simulink model "sim_3"  (R2015b)
settings: Solver=ode23  StartTime=0  StopTime=1200  FixedStep=1e-3  RelTol=1e-4
undefined symbols (not defined in the file or in its folder): alpha_nc, alpha_nw, angle_AW, angle_current, angle_SW, currentCoeffMatrix, f, Kd_surge, Kd_sway, Kd_yaw, Ki_surge, Ki_sway, Ki_yaw, Kp_surge, Kp_sway, Kp_yaw, mu, mu_SW, N_freq, Par, phi, S, Sim, T_pinv, TA_sampling_time, thrusterPositionX, thrusterPositionY, thrusters, thrustersInitialAlpha, U_mean_AW, U_mean_c, U_mean_w, V_c, windCoeffMatrix
libraries: simulink_extras x5, simulink x5, marine_gnc x2
settings Model: Creator=torstebo  LastModifiedBy=ShivJeet
settings SolverCC: MaxConsecutiveMinStep=3  SolverJacobianMethodControl=FullPerturbation  ZeroCrossControl=DisableAll  ZeroCrossAlgorithm=Adaptive
settings DataIOCC: Decimation=10  InitialState=xFinal  LimitDataPoints=off  SaveFormat=StructureWithTime  SaveOutput=off  InspectSignalLogs=on  VisualizeSimOutput=off  SaveTime=off
settings OptimizationCC: AccelVerboseBuild=on
settings DebuggingCC: AlgebraicLoopMsg=error  UnderspecifiedInitializationDetection=Classic  MergeDetectMultiDrivingBlocksExec=none  SolverPrmCheckMsg=warning  StateNameClashWarn=warning
settings HardwareCC: ProdBitPerPointer=32  ProdLargestAtomicFloat=None  ProdIntDivRoundTo=Undefined  ProdEndianess=Unspecified  ProdWordSize=32  ProdHWDeviceType=32-bit Generic
settings GRTTargetCC: GeneratePreprocessorConditionals=Disable all
settings ConfigComp: CovModelRefEnable=Off  CovSFcnEnable=off

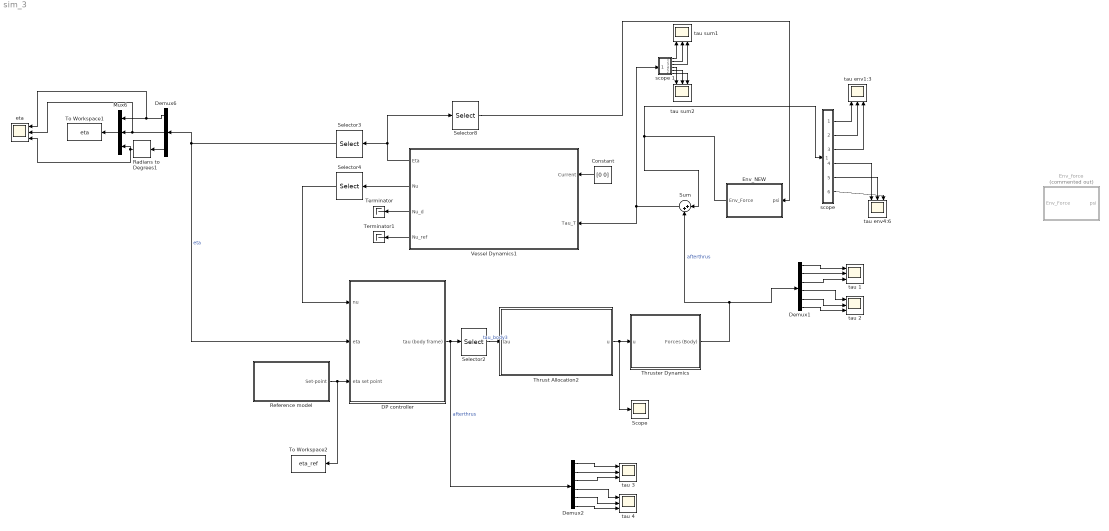
== system sim_3 ==
  Constant : Constant  Value=[0 0]
  DP controller : Subsystem
  Demux1 : Demux  Outputs=6
  Demux2 : Demux  Outputs=6
  Demux6 : Demux  Outputs=3
  Env_NEW : Subsystem
  Env_force : Subsystem  Commented=on
  Mux6 : Mux  Inputs=3
  Radians to Degrees1 : simulink_extras/Transformations/Radians to Degrees
  Reference model : Subsystem
  Scope : Scope
  Selector2 : Selector  InputPortWidth=6  IndexOptions=Index vector (dialog)  Indices=[1 2 6]  OutputSizes=1
  Selector3 : Selector  InputPortWidth=6  IndexOptions=Index vector (dialog)  Indices=[1 2 6]  OutputSizes=1
  Selector4 : Selector  InputPortWidth=6  IndexOptions=Index vector (dialog)  Indices=[1 2 6]  OutputSizes=1
  Selector8 : Selector  InputPortWidth=6  IndexOptions=Index vector (dialog)  Indices=[6]  OutputSizes=1
  Sum : Sum  Inputs=|++
  Terminator : Terminator
  Terminator1 : Terminator
  Thrust Allocation2 : Subsystem
  Thruster Dynamics : Subsystem  SystemSampleTime=TA_sampling_time  mask{wt=2, thrusterfault=off}
      mask prompts: wt "Thrusters Time constant"; thrusterfault "Thruster #3 fault?"
  To Workspace1 : ToWorkspace  VariableName=eta  SaveFormat=Timeseries  SampleTime=-1
  To Workspace2 : ToWorkspace  VariableName=eta_ref  SaveFormat=Timeseries  SampleTime=-1
  Vessel Dynamics1 : Subsystem
      mask Display:
      | image(imread('Files/supply.jpg'))
      | color('black'); port_label('output', 1, 'eta')
      | color('black'); port_label('output', 2, 'nu')
      | color('black'); port_label('output', 3, 'nu_d')
      | color('black'); port_label('output', 4, 'nu_ref')
      | color('black'); port_label('input', 1, 'nu_c')
      | color('black'); port_label('input', 2, 'tau')
  eta : Scope  NumInputPorts=3
  "scope " : Subsystem
  scope 1 : Subsystem
  tau {1..4} (4 alike) : Scope  NumInputPorts=3
  tau env1:3 : Scope  NumInputPorts=3
  tau env4:6 : Scope  NumInputPorts=3
  tau sum1 : Scope  NumInputPorts=3
  tau sum2 : Scope  NumInputPorts=3
  wires:
  Vessel Dynamics1/2(Nu) -> Selector4/1
  Constant/1 -> Vessel Dynamics1/1(Current)
  Reference model/1(Set-point) -> To Workspace2/1, DP controller/3(eta set point)
  Vessel Dynamics1/3(Nu_d) -> Terminator/1
  Thrust Allocation2/1(u) -> Scope/1, Thruster Dynamics/1(u)
  Selector4/1 -> DP controller/1(nu)
  Vessel Dynamics1/4(Nu_ref) -> Terminator1/1
  Thruster Dynamics/1(Forces (Body)) -> Sum/2, Demux1/1  "afterthrus"
  Selector3/1 -> Demux6/1, DP controller/2(eta)  "eta"
  Demux6/3 -> Radians to Degrees1/1
  Radians to Degrees1/1 -> Mux6/3, eta/3
  Demux6/2 -> eta/2, Mux6/2
  Demux6/1 -> Mux6/1, eta/1
  Mux6/1 -> To Workspace1/1
  Selector2/1 -> Thrust Allocation2/1(tau)  "tau_body3"
  Vessel Dynamics1/1(Eta) -> Selector3/1, Selector8/1
  Selector8/1 -> Env_NEW/1(psi)
  Sum/1 -> scope 1/1(In1), Vessel Dynamics1/2(Tau_T)
  Demux1/1 -> tau 1/1
  Demux1/2 -> tau 1/2
  Demux1/3 -> tau 1/3
  Demux1/4 -> tau 2/1
  Demux1/5 -> tau 2/2
  Demux1/6 -> tau 2/3
  Env_NEW/1(Env_Force) -> "scope "/1(In1), Sum/1
  "scope "/1(Out1) -> tau env1:3/1
  "scope "/3(Out3) -> tau env1:3/3
  "scope "/4(Out4) -> tau env4:6/1
  "scope "/5(Out5) -> tau env4:6/2
  "scope "/6(Out6) -> tau env4:6/3
  scope 1/1(Out1) -> tau sum1/1
  scope 1/2(Out2) -> tau sum1/2
  scope 1/3(Out3) -> tau sum1/3
  scope 1/4(Out4) -> tau sum2/1
  scope 1/5(Out5) -> tau sum2/2
  scope 1/6(Out6) -> tau sum2/3
  "scope "/2(Out2) -> tau env1:3/2
  DP controller/1(tau (body frame)) -> Demux2/1, Selector2/1  "afterthrus"
  Demux2/1 -> tau 3/1
  Demux2/2 -> tau 3/2
  Demux2/3 -> tau 3/3
  Demux2/4 -> tau 4/1
  Demux2/5 -> tau 4/2
  Demux2/6 -> tau 4/3

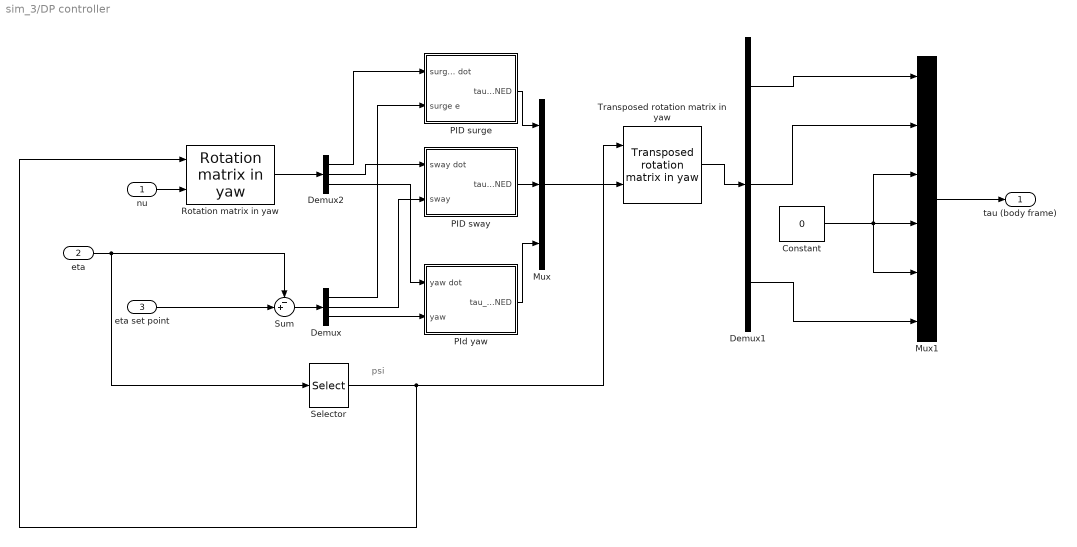
== system sim_3/DP controller ==
  note: psi
  nu : Inport
  eta : Inport  Port=2
  eta set point : Inport  Port=3
  Constant : Constant  Value=0
  Demux : Demux  Outputs=3
  Demux1 : Demux  Outputs=3
  Demux2 : Demux  Outputs=3
  Mux : Mux  Inputs=3
  Mux1 : Mux  Inputs=6
  PID surge : Subsystem
  PID sway : Subsystem
  "PId yaw " : Subsystem
  "Rotation matrix in yaw " : marine_gnc/Models/ Kinematics/Rotation matrix in yaw 
  Selector : Selector  InputPortWidth=3  IndexOptions=Index vector (dialog)  Indices=3  OutputSizes=1
  Sum : Sum  Inputs=-+|
  Transposed rotation matrix in yaw : marine_gnc/Models/ Kinematics/Transposed rotation  matrix in yaw
  tau (body frame) : Outport
  wires:
  Sum/1 -> Demux/1
  eta/1 -> Sum/1, Selector/1
  eta set point/1 -> Sum/2
  Demux2/1 -> PID surge/1(surge dot)
  Demux/1 -> PID surge/2(surge e)
  Demux2/2 -> PID sway/1(sway dot)
  Demux2/3 -> "PId yaw "/1(yaw dot)
  Demux/2 -> PID sway/2(sway)
  Demux/3 -> "PId yaw "/2(yaw)
  "PId yaw "/1(tau_yaw_NED) -> Mux/3
  PID surge/1(tau_surge_NED) -> Mux/1
  PID sway/1(tau_sway_NED) -> Mux/2
  nu/1 -> "Rotation matrix in yaw "/2
  Selector/1 -> Transposed rotation matrix in yaw/1, "Rotation matrix in yaw "/1
  "Rotation matrix in yaw "/1 -> Demux2/1
  Constant/1 -> Mux1/3, Mux1/4, Mux1/5
  Transposed rotation matrix in yaw/1 -> Demux1/1
  Demux1/1 -> Mux1/1
  Demux1/2 -> Mux1/2
  Demux1/3 -> Mux1/6
  Mux1/1 -> tau (body frame)/1
  ? -> ?
  Mux/1 -> Transposed rotation matrix in yaw/2

== system sim_3/Env_NEW ==
  psi : Inport
  Constant : Constant  Value=windCoeffMatrix
  Constant1 : Constant  Value=currentCoeffMatrix
  Current : Subsystem
  Product : Product  Inputs=3  RndMeth=Zero
  Product1 : Product  Inputs=3  RndMeth=Zero
  Radians to Degrees : simulink_extras/Transformations/Radians to Degrees
  Sum : Sum  Inputs=+-|
  Sum1 : Sum  Inputs=+|+
  Sum2 : Sum  Inputs=|+-
  Wind : Subsystem
  get current coeffcients : MATLAB Function  TreatAsAtomicUnit=on
  get wind coeffcients : MATLAB Function  TreatAsAtomicUnit=on
  Env_Force : Outport
  wires:
  Wind/1(Wind velocity) -> Product/2, Product/1
  Wind/2(Win direction) -> Sum/1
  psi/1 -> Radians to Degrees/1
  Sum1/1 -> Env_Force/1
  Current/1(current velocity) -> Product1/2, Product1/1
  Radians to Degrees/1 -> Sum/2, Sum2/2
  Current/2(current direction) -> Sum2/1
  Sum2/1 -> get current coeffcients/1(alpha)
  get current coeffcients/1(C) -> Product1/3
  Sum/1 -> get wind coeffcients/1(alpha)
  get wind coeffcients/1(C) -> Product/3
  Product1/1 -> Sum1/2
  Product/1 -> Sum1/1
  Constant/1 -> get wind coeffcients/2(windCoeffMatrix)
  Constant1/1 -> get current coeffcients/2(currentCoeffMatrix)

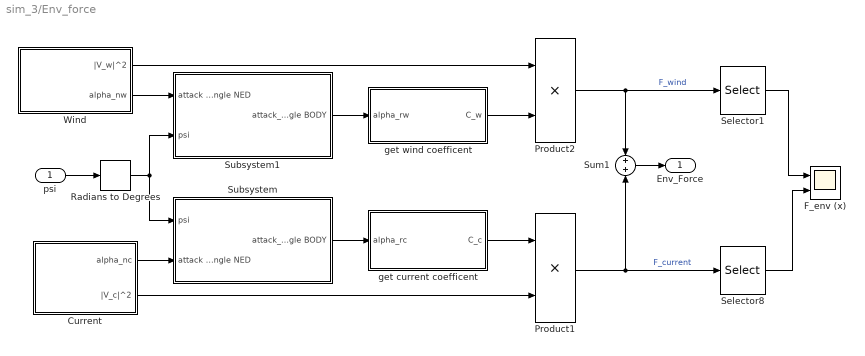
== system sim_3/Env_force ==
  psi : Inport
  "Current " : Subsystem
  F_env (x) : Scope  NumInputPorts=2
  Product1 : Product  RndMeth=Zero
  Product2 : Product  RndMeth=Zero
  Radians to Degrees : simulink_extras/Transformations/Radians to Degrees
  Selector1 : Selector  InputPortWidth=6  IndexOptions=Index vector (dialog)  Indices=[2]  OutputSizes=1
  Selector8 : Selector  InputPortWidth=6  IndexOptions=Index vector (dialog)  Indices=[2]  OutputSizes=1
  Subsystem : Subsystem
  Subsystem1 : Subsystem
  Sum1 : Sum  Inputs=+|+
  Wind : Subsystem
  "get current coefficent " : MATLAB Function  TreatAsAtomicUnit=on
  "get wind coefficent " : MATLAB Function  TreatAsAtomicUnit=on
  Env_Force : Outport
  wires:
  Wind/1(|V_w|^2) -> Product2/1
  psi/1 -> Radians to Degrees/1
  Sum1/1 -> Env_Force/1
  Product2/1 -> Selector1/1, Sum1/1  "F_wind"
  "Current "/2(|V_c|^2) -> Product1/2
  Product1/1 -> Selector8/1, Sum1/2  "F_current"
  Selector1/1 -> F_env (x)/1
  Selector8/1 -> F_env (x)/2
  "get current coefficent "/1(C_c) -> Product1/1
  Subsystem/1(attack_angle BODY) -> "get current coefficent "/1(alpha_rc)
  Radians to Degrees/1 -> Subsystem/1(psi), Subsystem1/2(psi)
  "Current "/1(alpha_nc) -> Subsystem/2(attack angle NED)
  Wind/2(alpha_nw) -> Subsystem1/1(attack angle NED)
  Subsystem1/1(attack_angle BODY) -> "get wind coefficent "/1(alpha_rw)
  "get wind coefficent "/1(C_w) -> Product2/2

== system sim_3/Reference model ==
  Mux : Mux  Inputs=3
  Sp_surge : Constant  Value=10*1  VectorParams1D=off
  Sp_sway : Constant  Value=2*1
  Sp_yaw : Constant  Value=pi/2*1
  Transfer Fcn1 : TransferFcn  Numerator=[0.05]  Denominator=[1 0.05]
  Transfer Fcn2 : TransferFcn  Numerator=[0.01]  Denominator=[1 0.01]
  Transfer Fcn3 : TransferFcn  Numerator=[0.05]  Denominator=[1 0.05]
  Set-point : Outport
  wires:
  Mux/1 -> Set-point/1
  Transfer Fcn1/1 -> Mux/1
  Transfer Fcn2/1 -> Mux/2
  Transfer Fcn3/1 -> Mux/3
  Sp_surge/1 -> Transfer Fcn1/1
  Sp_sway/1 -> Transfer Fcn2/1
  Sp_yaw/1 -> Transfer Fcn3/1

== system sim_3/Thrust Allocation2 ==
  tau : Inport
  Gain : Gain  Gain=T_pinv  Multiplication=Matrix(K*u) (u vector)
  u : Outport
  wires:
  tau/1 -> Gain/1
  Gain/1 -> u/1

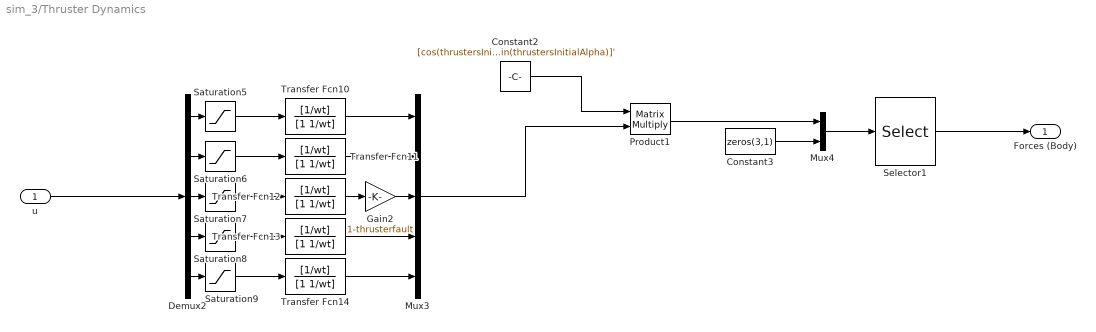
== system sim_3/Thruster Dynamics ==
  u : Inport  PortDimensions=[5 1]
  Constant2 : Constant  Value=[cos(thrustersInitialAlpha) sin(thrustersInitialAlpha) -thrusterPositionY.*cos(thrustersInitialAlpha)+thrusterPositionX.*sin(thrustersInitialAlpha)]'
  Constant3 : Constant  Value=zeros(3,1)
  Demux2 : Demux  Outputs=5
  Gain2 : Gain  Gain=1-thrusterfault
  Mux3 : Mux  Inputs=5
  Mux4 : Mux  Inputs=2
  Product1 : Product  Multiplication=Matrix(*)
  Saturation5 : Saturate  UpperLimit=thrusters(1).rated_thrust  LowerLimit=-thrusters(1).rated_thrust
  Saturation6 : Saturate  UpperLimit=thrusters(2).rated_thrust  LowerLimit=-thrusters(2).rated_thrust
  Saturation7 : Saturate  UpperLimit=thrusters(3).rated_thrust  LowerLimit=-thrusters(3).rated_thrust
  Saturation8 : Saturate  UpperLimit=thrusters(4).rated_thrust  LowerLimit=-thrusters(4).rated_thrust
  Saturation9 : Saturate  UpperLimit=thrusters(5).rated_thrust  LowerLimit=-thrusters(5).rated_thrust
  Selector1 : Selector  InputPortWidth=6  IndexOptions=Index vector (dialog)  Indices=[1 2 4 5 6 3]  OutputSizes=1
  Transfer Fcn{10..14} (5 alike) : TransferFcn  Numerator=[1/wt]  Denominator=[1 1/wt]
  Forces (Body) : Outport
  wires:
  Selector1/1 -> Forces (Body)/1
  Constant2/1 -> Product1/1
  Product1/1 -> Mux4/1
  Saturation5/1 -> Transfer Fcn10/1
  Demux2/1 -> Saturation5/1
  Demux2/2 -> Saturation6/1
  Saturation6/1 -> Transfer Fcn11/1
  Demux2/3 -> Saturation7/1
  Saturation7/1 -> Transfer Fcn12/1
  Demux2/4 -> Saturation8/1
  Saturation8/1 -> Transfer Fcn13/1
  Demux2/5 -> Saturation9/1
  Saturation9/1 -> Transfer Fcn14/1
  u/1 -> Demux2/1
  Transfer Fcn10/1 -> Mux3/1
  Transfer Fcn11/1 -> Mux3/2
  Transfer Fcn12/1 -> Gain2/1
  Transfer Fcn13/1 -> Mux3/4
  Transfer Fcn14/1 -> Mux3/5
  Mux4/1 -> Selector1/1
  Constant3/1 -> Mux4/2
  Gain2/1 -> Mux3/3
  Mux3/1 -> Product1/2

== system sim_3/Vessel Dynamics1 ==
  note: VESSEL MODULE
      | Consists of a WF and a LF module, which may be enabled or disabled in the Parameters file.
      | The LF and WFmotion components are written to the workspace for processing, and added for
      | use in the simulator.
  Current : Inport
  Tau_T : Inport  Port=2
  Vessel LF 6DOF : Subsystem
  Eta : Outport
  Nu : Outport  Port=2
  Nu_d : Outport  Port=3
  Nu_ref : Outport  Port=4
  wires:
  Current/1 -> Vessel LF 6DOF/2(Current_NED)
  Tau_T/1 -> Vessel LF 6DOF/1(External forces)  "Tau_T"
  Vessel LF 6DOF/1(Eta) -> Eta/1  "Eta_LF"
  Vessel LF 6DOF/2(Nu) -> Nu/1  "Nu_LF"
  Vessel LF 6DOF/3(Nu_d) -> Nu_d/1
  Vessel LF 6DOF/4(Nu_r) -> Nu_ref/1

== system sim_3/scope  ==
  In1 : Inport
  Demux2 : Demux  Outputs=6
  Out1 : Outport
  Out2 : Outport  Port=2
  Out3 : Outport  Port=3
  Out4 : Outport  Port=4
  Out5 : Outport  Port=5
  Out6 : Outport  Port=6
  wires:
  Demux2/2 -> Out2/1
  Demux2/1 -> Out1/1
  Demux2/5 -> Out5/1
  Demux2/4 -> Out4/1
  Demux2/6 -> Out6/1
  Demux2/3 -> Out3/1
  In1/1 -> Demux2/1

== system sim_3/scope 1 ==
  In1 : Inport
  Demux2 : Demux  Outputs=6
  Out1 : Outport
  Out2 : Outport  Port=2
  Out3 : Outport  Port=3
  Out4 : Outport  Port=4
  Out5 : Outport  Port=5
  Out6 : Outport  Port=6
  wires:
  Demux2/2 -> Out2/1
  Demux2/1 -> Out1/1
  Demux2/5 -> Out5/1
  Demux2/4 -> Out4/1
  Demux2/6 -> Out6/1
  Demux2/3 -> Out3/1
  In1/1 -> Demux2/1

== system sim_3/DP controller/PID surge ==
  surge dot : Inport
  surge e : Inport  Port=2
  Gain2 : Gain  Gain=Ki_surge
  Integrator : Integrator
  KP : Gain  Gain=Kp_surge
  Kd : Gain  Gain=Kd_surge
  Sum : Sum  Inputs=|-++
  tau_surge_NED : Outport
  wires:
  surge dot/1 -> Kd/1
  surge e/1 -> KP/1, Integrator/1
  Integrator/1 -> Gain2/1
  Kd/1 -> Sum/1
  KP/1 -> Sum/2
  Gain2/1 -> Sum/3
  Sum/1 -> tau_surge_NED/1

== system sim_3/DP controller/PID sway ==
  sway dot : Inport
  sway : Inport  Port=2
  Integrator : Integrator
  Kd : Gain  Gain=Kd_sway
  Ki : Gain  Gain=Ki_sway
  Kp : Gain  Gain=Kp_sway
  Sum : Sum  Inputs=|-++
  tau_sway_NED : Outport
  wires:
  sway dot/1 -> Kd/1
  sway/1 -> Kp/1, Integrator/1
  Integrator/1 -> Ki/1
  Kd/1 -> Sum/1
  Kp/1 -> Sum/2
  Ki/1 -> Sum/3
  Sum/1 -> tau_sway_NED/1

== system sim_3/DP controller/PId yaw  ==
  yaw dot : Inport
  yaw : Inport  Port=2
  Gain : Gain  Gain=Kd_yaw
  Gain1 : Gain  Gain=Kp_yaw
  Gain2 : Gain  Gain=Ki_yaw
  Integrator : Integrator
  Sum : Sum  Inputs=|-++
  tau_yaw_NED : Outport
  wires:
  yaw dot/1 -> Gain/1
  yaw/1 -> Gain1/1, Integrator/1
  Integrator/1 -> Gain2/1
  Gain/1 -> Sum/1
  Gain1/1 -> Sum/2
  Gain2/1 -> Sum/3
  Sum/1 -> tau_yaw_NED/1

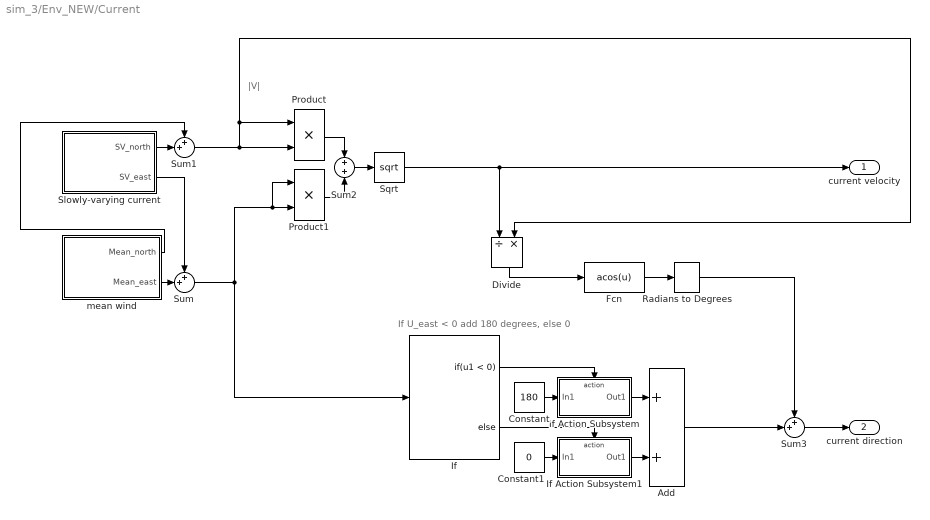
== system sim_3/Env_NEW/Current ==
  note: If U_east < 0 add 180 degrees, else 0
  note: |V|
  Add : Sum
  Constant : Constant  Value=180
  Constant1 : Constant  Value=0
  Divide : Product  Inputs=/*
  Fcn : Fcn  Expr=acos(u)
  "If " : If  IfExpression=u1 < 0
  If Action Subsystem : Subsystem  TreatAsAtomicUnit=on
  If Action Subsystem1 : Subsystem  TreatAsAtomicUnit=on
  Product : Product
  Product1 : Product
  Radians to Degrees : simulink_extras/Transformations/Radians to Degrees
  Slowly-varying current : Subsystem
  Sqrt : Sqrt  SaturateOnIntegerOverflow=on
  Sum : Sum  Inputs=++|
  Sum1 : Sum  Inputs=++|
  Sum2 : Sum  Inputs=+|+
  Sum3 : Sum  Inputs=++|
  mean wind : Subsystem
  current velocity : Outport
  current direction : Outport  Port=2
  wires:
  Slowly-varying current/1(SV_north) -> Sum1/2
  Slowly-varying current/2(SV_east) -> Sum/1
  mean wind/2(Mean_east) -> Sum/2
  Divide/1 -> Fcn/1
  Fcn/1 -> Radians to Degrees/1
  Sum3/1 -> current direction/1
  Radians to Degrees/1 -> Sum3/1
  If Action Subsystem/1(Out1) -> Add/1
  Add/1 -> Sum3/2
  mean wind/1(Mean_north) -> Sum1/1
  Sum1/1 -> Product/2, Product/1, Divide/2
  Sum/1 -> Product1/1, Product1/2, "If "/1
  Product/1 -> Sum2/1
  Product1/1 -> Sum2/2
  Sum2/1 -> Sqrt/1
  Sqrt/1 -> Divide/1, current velocity/1
  Constant/1 -> If Action Subsystem/1(In1)
  "If "/1 -> If Action Subsystem/Action
  "If "/2 -> If Action Subsystem1/Action
  Constant1/1 -> If Action Subsystem1/1(In1)
  If Action Subsystem1/1(Out1) -> Add/2

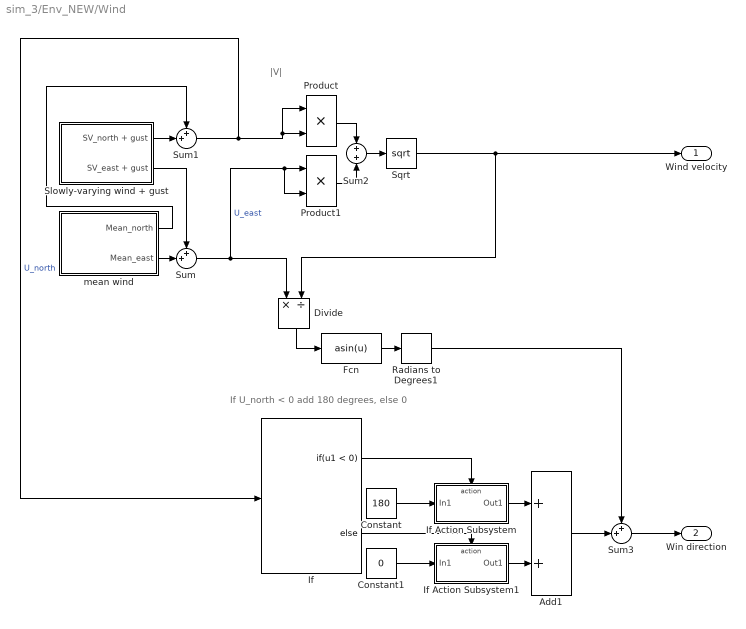
== system sim_3/Env_NEW/Wind ==
  note: |V|
  note: If U_north < 0 add 180 degrees, else 0
  Add1 : Sum
  Constant : Constant  Value=180
  Constant1 : Constant  Value=0
  Divide : Product  Inputs=*/
  Fcn : Fcn  Expr=asin(u)
  If : If  IfExpression=u1 < 0
  If Action Subsystem : Subsystem  TreatAsAtomicUnit=on
  If Action Subsystem1 : Subsystem  TreatAsAtomicUnit=on
  Product : Product
  Product1 : Product
  Radians to Degrees1 : simulink_extras/Transformations/Radians to Degrees
  Slowly-varying wind + gust : Subsystem
  Sqrt : Sqrt  SaturateOnIntegerOverflow=on
  Sum : Sum  Inputs=++|
  Sum1 : Sum  Inputs=++|
  Sum2 : Sum  Inputs=+|+
  Sum3 : Sum  Inputs=++|
  mean wind : Subsystem
  Wind velocity : Outport
  Win direction : Outport  Port=2
  wires:
  Slowly-varying wind + gust/2(SV_east + gust) -> Sum/1
  mean wind/2(Mean_east) -> Sum/2
  Sum1/1 -> Product/1, Product/2, If/1  "U_north"
  Sum/1 -> Product1/2, Product1/1, Divide/1  "U_east"
  Sqrt/1 -> Divide/2, Wind velocity/1
  Slowly-varying wind + gust/1(SV_north + gust) -> Sum1/2
  mean wind/1(Mean_north) -> Sum1/1
  Product/1 -> Sum2/1
  Product1/1 -> Sum2/2
  Sum2/1 -> Sqrt/1
  Divide/1 -> Fcn/1
  Fcn/1 -> Radians to Degrees1/1
  Radians to Degrees1/1 -> Sum3/1
  Add1/1 -> Sum3/2
  Sum3/1 -> Win direction/1
  If Action Subsystem/1(Out1) -> Add1/1
  Constant/1 -> If Action Subsystem/1(In1)
  If/1 -> If Action Subsystem/Action
  If/2 -> If Action Subsystem1/Action
  Constant1/1 -> If Action Subsystem1/1(In1)
  If Action Subsystem1/1(Out1) -> Add1/2

== system sim_3/Env_force/Current  ==
  Product : Product
  alpha current : Constant  Value=angle_current
  current speed : Constant  Value=V_c
  alpha_nc : Outport
  |V_c|^2 : Outport  Port=2
  wires:
  current speed/1 -> Product/2, Product/1
  alpha current/1 -> alpha_nc/1
  Product/1 -> |V_c|^2/1

== system sim_3/Env_force/Subsystem ==
  psi : Inport
  attack angle NED : Inport  Port=2
  Constant1 : Constant  Value=180
  Sum1 : Sum  Inputs=++-|
  attack_angle BODY : Outport
  wires:
  attack angle NED/1 -> Sum1/3
  Constant1/1 -> Sum1/1
  Sum1/1 -> attack_angle BODY/1
  psi/1 -> Sum1/2

== system sim_3/Env_force/Subsystem1 ==
  attack angle NED : Inport
  psi : Inport  Port=2
  Constant : Constant  Value=180
  Sum2 : Sum  Inputs=++-|
  attack_angle BODY : Outport
  wires:
  attack angle NED/1 -> Sum2/3
  Constant/1 -> Sum2/1
  Sum2/1 -> attack_angle BODY/1
  psi/1 -> Sum2/2

== system sim_3/Env_force/Wind ==
  Divide : Product  Inputs=/*
  Product : Product
  Slowly-varying wind : Subsystem
  Sum : Sum  Inputs=|++
  Sum1 : Sum  Inputs=++|
  average wind : Subsystem
  |V_w|^2 : Outport
  alpha_nw : Outport  Port=2
  wires:
  Slowly-varying wind/1(U_sv) -> Sum/1
  Sum/1 -> Product/1, Divide/1, Product/2
  Sum1/1 -> Divide/2
  Divide/1 -> alpha_nw/1
  average wind/2(wheigted direction) -> Sum1/1
  Slowly-varying wind/2(weigthed direction) -> Sum1/2
  average wind/1(speed) -> Sum/2
  Product/1 -> |V_w|^2/1

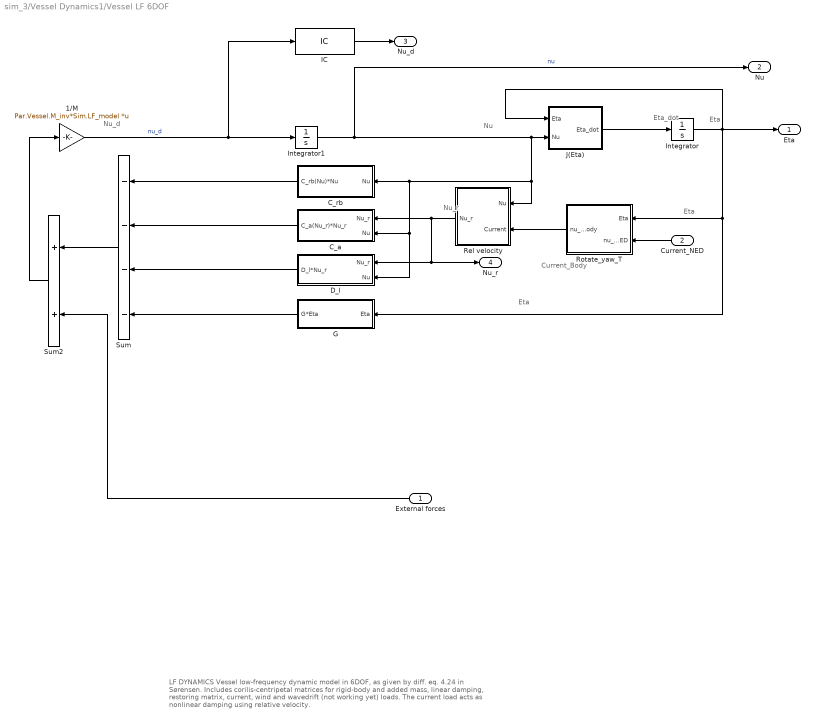
== system sim_3/Vessel Dynamics1/Vessel LF 6DOF ==
  note: Nu_d
  note: Nu
  note: Eta
  note: Current_Body
  note: Eta
  note: Nu_r
  note: Eta
  note: LF DYNAMICS
      | Vessel low-frequency dynamic model in 6DOF, as given by diff. eq. 4.24 in Sørensen.
      | Includes corilis-centripetal matrices for rigid-body and added mass, linear damping,
      | restoring matrix, current, wind and wavedrift (not working yet) loads. The current load
      | acts as nonlinear damping using relative velocity.
  note: Eta_dot
  External forces : Inport
  Current_NED : Inport  Port=2
  1/M : Gain  Gain=Par.Vessel.M_inv*Sim.LF_model  Multiplication=Matrix(K*u) (u vector)  SaturateOnIntegerOverflow=on  OutDataTypeStr=Inherit: Same as input  ParamDataTypeStr=Inherit: Same as input
  C_a : Subsystem
  C_rb : Subsystem
  D_l : Subsystem
      settings: MinAlgLoopOccurrences=on
  G : Subsystem
  IC : InitialCondition  Value=Sim.Nu_d_init
  Integrator : Integrator  InitialCondition=Sim.Eta_init
  Integrator1 : Integrator  InitialCondition=Sim.Nu_init
  J(Eta) : Subsystem
  Rel velocity : Subsystem
  Rotate_yaw_T : Subsystem
  Sum : Sum  Inputs=----  SaturateOnIntegerOverflow=on
  Sum2 : Sum  SaturateOnIntegerOverflow=on
  Eta : Outport
  Nu : Outport  Port=2
  Nu_d : Outport  Port=3
  Nu_r : Outport  Port=4
  wires:
  1/M/1 -> IC/1, Integrator1/1  "nu_d"
  J(Eta)/1(Eta_dot) -> Integrator/1
  Integrator/1 -> J(Eta)/1(Eta), Eta/1, Rotate_yaw_T/1(Eta), G/1(Eta)
  Integrator1/1 -> Nu/1, J(Eta)/2(Nu), Rel velocity/1(Nu), C_a/2(Nu), D_l/2(Nu), C_rb/1(Nu)  "nu"
  Current_NED/1 -> Rotate_yaw_T/2(nu_2D_NED)
  Rotate_yaw_T/1(nu_2D_body) -> Rel velocity/2(Current)
  Rel velocity/1(Nu_r) -> D_l/1(Nu_r), Nu_r/1, C_a/1(Nu_r)
  Sum/1 -> Sum2/1
  External forces/1 -> Sum2/2
  Sum2/1 -> 1/M/1
  C_rb/1(C_rb(Nu)*Nu) -> Sum/1
  C_a/1(C_a(Nu_r)*Nu_r) -> Sum/2
  D_l/1(D_l*Nu_r) -> Sum/3
  G/1(G*Eta) -> Sum/4
  IC/1 -> Nu_d/1

== system sim_3/Env_NEW/Current/If Action Subsystem ==
  In1 : Inport
  Action Port : ActionPort  ActionType=then
  Out1 : Outport
  wires:
  In1/1 -> Out1/1

== system sim_3/Env_NEW/Current/If Action Subsystem1 ==
  In1 : Inport
  Action Port : ActionPort  ActionType=else
  Out1 : Outport
  wires:
  In1/1 -> Out1/1

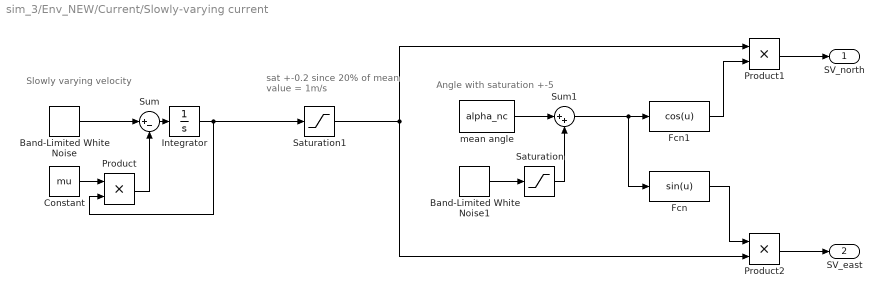
== system sim_3/Env_NEW/Current/Slowly-varying current ==
  note: Angle with saturation +-5
  note: Slowly varying velocity
  note: sat +-0.2 since 20%
      | of mean value = 1m/s
  Band-Limited White Noise : simulink/Sources/Band-Limited White Noise  Cov=[0.00005]  Ts=20  seed=[23343]
  Band-Limited White Noise1 : simulink/Sources/Band-Limited White Noise  Cov=[0.00005]  Ts=20  seed=[23344]
  Constant : Constant  Value=mu
  Fcn : Fcn  Expr=sin(u)
  Fcn1 : Fcn  Expr=cos(u)
  Integrator : Integrator
  Product : Product  RndMeth=Zero
  Product1 : Product  RndMeth=Zero
  Product2 : Product  RndMeth=Zero
  Saturation : Saturate  UpperLimit=(5*pi)/180  LowerLimit=-(5*pi)/180
  Saturation1 : Saturate  UpperLimit=0.2  LowerLimit=-0.2
  Sum : Sum  Inputs=|+-
  Sum1 : Sum  Inputs=|++
  mean angle : Constant  Value=alpha_nc
  SV_north : Outport
  SV_east : Outport  Port=2
  wires:
  Band-Limited White Noise/1 -> Sum/1
  Sum/1 -> Integrator/1
  Integrator/1 -> Product/2, Saturation1/1
  Product/1 -> Sum/2
  Constant/1 -> Product/1
  Fcn1/1 -> Product1/2
  mean angle/1 -> Sum1/1
  Sum1/1 -> Fcn/1, Fcn1/1
  Saturation/1 -> Sum1/2
  Band-Limited White Noise1/1 -> Saturation/1
  Product1/1 -> SV_north/1
  Product2/1 -> SV_east/1
  Saturation1/1 -> Product2/2, Product1/1
  Fcn/1 -> Product2/1

== system sim_3/Env_NEW/Current/mean wind ==
  Constant : Constant  Value=U_mean_c
  Fcn : Fcn  Expr=sin(u)
  Fcn1 : Fcn  Expr=cos(u)
  Product1 : Product  RndMeth=Zero
  Product2 : Product  RndMeth=Zero
  meen wind : Constant  Value=alpha_nc
  Mean_north : Outport
  Mean_east : Outport  Port=2
  wires:
  Constant/1 -> Product1/1, Product2/2
  Fcn1/1 -> Product1/2
  Product1/1 -> Mean_north/1
  Product2/1 -> Mean_east/1
  meen wind/1 -> Fcn/1, Fcn1/1
  Fcn/1 -> Product2/1

== system sim_3/Env_NEW/Wind/If Action Subsystem ==
  In1 : Inport
  Action Port : ActionPort  ActionType=then
  Out1 : Outport
  wires:
  In1/1 -> Out1/1

== system sim_3/Env_NEW/Wind/If Action Subsystem1 ==
  In1 : Inport
  Action Port : ActionPort  ActionType=else
  Out1 : Outport
  wires:
  In1/1 -> Out1/1

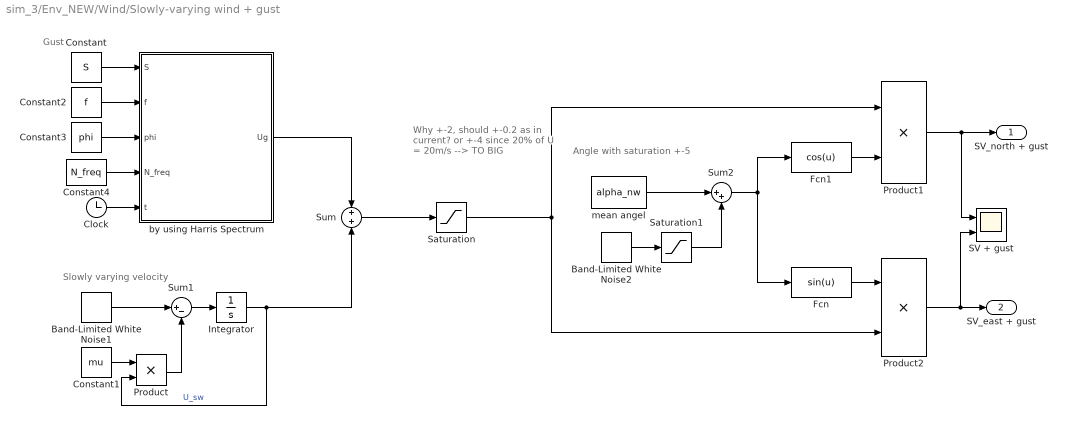
== system sim_3/Env_NEW/Wind/Slowly-varying wind + gust ==
  note: Gust
  note: Slowly varying velocity
  note: Angle with saturation +-5
  note: Why +-2, should
      | +-0.2 as in current?
      | or +-4 since 20% of
      | U = 20m/s --> TO BIG
  Band-Limited White Noise1 : simulink/Sources/Band-Limited White Noise  Cov=[0.005]  Ts=20  seed=[23341]
  Band-Limited White Noise2 : simulink/Sources/Band-Limited White Noise  Cov=[0.005]  Ts=20  seed=[23342]
  Clock : Clock
  Constant : Constant  Value=S
  Constant1 : Constant  Value=mu
  Constant2 : Constant  Value=f
  Constant3 : Constant  Value=phi
  Constant4 : Constant  Value=N_freq
  Fcn : Fcn  Expr=sin(u)
  Fcn1 : Fcn  Expr=cos(u)
  Integrator : Integrator
  Product : Product  RndMeth=Zero
  Product1 : Product  RndMeth=Zero
  Product2 : Product  RndMeth=Zero
  SV + gust : Scope  NumInputPorts=2
  Saturation : Saturate  UpperLimit=2  LowerLimit=-2
  Saturation1 : Saturate  UpperLimit=(5*pi)/180  LowerLimit=-(5*pi)/180
  Sum : Sum  Inputs=+|+
  Sum1 : Sum  Inputs=|+-
  Sum2 : Sum  Inputs=|++
  by using Harris Spectrum : MATLAB Function  TreatAsAtomicUnit=on  SystemSampleTime=1
  mean angel : Constant  Value=alpha_nw
  SV_north + gust : Outport
  SV_east + gust : Outport  Port=2
  wires:
  Fcn1/1 -> Product1/2
  Product1/1 -> SV + gust/1, SV_north + gust/1
  Product2/1 -> SV_east + gust/1, SV + gust/2
  Sum2/1 -> Fcn/1, Fcn1/1
  Integrator/1 -> Sum/2, Product/2  "U_sw"
  Saturation/1 -> Product1/1, Product2/2
  Constant1/1 -> Product/1
  Sum1/1 -> Integrator/1
  Product/1 -> Sum1/2
  Band-Limited White Noise1/1 -> Sum1/1
  mean angel/1 -> Sum2/1
  Saturation1/1 -> Sum2/2
  Band-Limited White Noise2/1 -> Saturation1/1
  Fcn/1 -> Product2/1
  Constant/1 -> by using Harris Spectrum/1(S)
  Constant2/1 -> by using Harris Spectrum/2(f)
  Constant3/1 -> by using Harris Spectrum/3(phi)
  Constant4/1 -> by using Harris Spectrum/4(N_freq)
  Clock/1 -> by using Harris Spectrum/5(t)
  Sum/1 -> Saturation/1
  by using Harris Spectrum/1(Ug) -> Sum/1

== system sim_3/Env_NEW/Wind/mean wind ==
  Constant : Constant  Value=U_mean_w
  Fcn : Fcn  Expr=sin(u)
  Fcn1 : Fcn  Expr=cos(u)
  Product1 : Product  RndMeth=Zero
  Product2 : Product  RndMeth=Zero
  mean wind : Constant  Value=alpha_nw
  Mean_north : Outport
  Mean_east : Outport  Port=2
  wires:
  Constant/1 -> Product2/2, Product1/1
  Fcn1/1 -> Product1/2
  Product1/1 -> Mean_north/1
  mean wind/1 -> Fcn1/1, Fcn/1
  Fcn/1 -> Product2/1
  Product2/1 -> Mean_east/1

== system sim_3/Env_force/Wind/Slowly-varying wind ==
  " angle SW" : Constant  Value=angle_SW
  Band-Limited White Noise : simulink/Sources/Band-Limited White Noise  Cov=white_noise_power_SW  Ts=1  seed=[23341]
  Constant : Constant  Value=mu_SW
  Integrator : Integrator
  Product : Product  RndMeth=Zero
  Product1 : Product  RndMeth=Zero
  Sum : Sum  Inputs=|+-
  U_sv : Outport
  weigthed direction : Outport  Port=2
  wires:
  Band-Limited White Noise/1 -> Sum/1
  Sum/1 -> Integrator/1
  Integrator/1 -> Product/2, U_sv/1, Product1/1
  Product/1 -> Sum/2
  Constant/1 -> Product/1
  Product1/1 -> weigthed direction/1
  " angle SW"/1 -> Product1/2

== system sim_3/Env_force/Wind/average wind ==
  Product : Product  RndMeth=Zero
  U_mean : Constant  Value=U_mean_AW
  wind angle : Constant  Value=angle_AW
  speed : Outport
  wheigted direction : Outport  Port=2
  wires:
  U_mean/1 -> speed/1, Product/1
  wind angle/1 -> Product/2
  Product/1 -> wheigted direction/1

== system sim_3/Vessel Dynamics1/Vessel LF 6DOF/C_a ==
  note: C_a
      | Coriolis-centripetal added mass force calculation using the S-function m2c_S.
      | This effect can be included/excluded from the Parameters file.
      | A choice of using absolute or relative vessel velocity is also given.
      | OS2002
  Nu_r : Inport
  Nu : Inport  Port=2
  C_a calculation : Subsystem  TreatAsAtomicUnit=on
  Enable Coriolis added mass force : Constant  Value=Sim.C_a
  Sim.Nu_r_C_a : Constant  Value=Sim.Nu_r_C_a
  Switch : Switch  Criteria=u2 > Threshold  SaturateOnIntegerOverflow=on
  C_a(Nu_r)*Nu_r : Outport
  wires:
  C_a calculation/1(F) -> C_a(Nu_r)*Nu_r/1
  Nu_r/1 -> Switch/1
  Nu/1 -> Switch/3
  Sim.Nu_r_C_a/1 -> Switch/2
  Switch/1 -> C_a calculation/1(Nu_r)
  Enable Coriolis added mass force/1 -> C_a calculation/Enable

== system sim_3/Vessel Dynamics1/Vessel LF 6DOF/C_rb ==
  note: C_rb
      | Coriolis-centripetal rigid-body force calculation using the S-function m2c_S.
      | This effect can be included/excluded from the Parameters file.
      | OS2002
  Nu : Inport
  C_rb Calculation : Subsystem  TreatAsAtomicUnit=on
  Enable Coriolis added mass force : Constant  Value=Sim.C_rb
  C_rb(Nu)*Nu : Outport
  wires:
  Nu/1 -> C_rb Calculation/1(Nu_r)
  Enable Coriolis added mass force/1 -> C_rb Calculation/Enable
  C_rb Calculation/1(F) -> C_rb(Nu)*Nu/1

== system sim_3/Vessel Dynamics1/Vessel LF 6DOF/D_l ==
  note: D_l
      | Linear damping, matrix formulation.
      | This effect can be included/excluded from the Parameters file.
      | A choice of using absolute or relative vessel velocity is also given.
      | OS2002
  Nu_r : Inport
  Nu : Inport  Port=2
  D_l : Gain  Gain=Par.Vessel.DL  Multiplication=Matrix(K*u)  SaturateOnIntegerOverflow=on  OutDataTypeStr=Inherit: Same as input  ParamDataTypeStr=Inherit: Same as input
  Include D_l : Gain  Gain=Sim.D_l  SaturateOnIntegerOverflow=on  OutDataTypeStr=Inherit: Same as input  ParamDataTypeStr=Inherit: Same as input
  Sim.Nu_r_D_l : Constant  Value=Sim.Nu_r_D_l
  Switch : Switch  Criteria=u2 > Threshold  SaturateOnIntegerOverflow=on
  D_l*Nu_r : Outport
  wires:
  D_l/1 -> Include D_l/1
  Include D_l/1 -> D_l*Nu_r/1
  Switch/1 -> D_l/1
  Nu_r/1 -> Switch/1
  Nu/1 -> Switch/3
  Sim.Nu_r_D_l/1 -> Switch/2

== system sim_3/Vessel Dynamics1/Vessel LF 6DOF/G ==
  note: G
      | Standard restoring matrix. This effect can
      | be included/excluded from the Parameters file.
      | OS2002
  Eta : Inport
  G : Gain  Gain=Par.Vessel.G  Multiplication=Matrix(K*u)  SaturateOnIntegerOverflow=on  OutDataTypeStr=Inherit: Same as input  ParamDataTypeStr=Inherit: Same as input
  Include G : Gain  Gain=Sim.G  SaturateOnIntegerOverflow=on  OutDataTypeStr=Inherit: Same as input  ParamDataTypeStr=Inherit: Same as input
  G*Eta : Outport
  wires:
  Eta/1 -> G/1
  G/1 -> Include G/1
  Include G/1 -> G*Eta/1

== system sim_3/Vessel Dynamics1/Vessel LF 6DOF/J(Eta) ==
  note: Theta
  note: v
  note: omega
  note: J(Eta)
      | Standard 6DOF rotation matrix, as defined by Fossen. Using the two
      | rotation matrices Rnb and Tnb from the gnc Simulink toolbox.
      | OS2002
  Eta : Inport
  Nu : Inport  Port=2
  Mux : Mux  Inputs=2
  Product : Product  Inputs=**  Multiplication=Matrix(*)  SaturateOnIntegerOverflow=on  OutDataTypeStr=Inherit: Same as first input
  Product1 : Product  Inputs=**  Multiplication=Matrix(*)  SaturateOnIntegerOverflow=on  OutDataTypeStr=Inherit: Same as first input
  Rnb_gnc : Subsystem
  Selector : Selector  InputPortWidth=6  IndexOptions=Index vector (dialog)  Indices=[4 5 6]  OutputSizes=1
  Selector1 : Selector  InputPortWidth=6  IndexOptions=Index vector (dialog)  Indices=[1 2 3]  OutputSizes=1
  Selector2 : Selector  InputPortWidth=6  IndexOptions=Index vector (dialog)  Indices=[4 5 6]  OutputSizes=1
  Tnb_gnc : Subsystem
  Eta_dot : Outport
  wires:
  Selector/1 -> Tnb_gnc/1(theta), Rnb_gnc/1(theta)
  Eta/1 -> Selector/1
  Rnb_gnc/1(Rzyx) -> Product/1
  Nu/1 -> Selector1/1, Selector2/1
  Selector1/1 -> Product/2
  Selector2/1 -> Product1/2
  Tnb_gnc/1(T) -> Product1/1
  Product/1 -> Mux/1
  Mux/1 -> Eta_dot/1
  Product1/1 -> Mux/2

== system sim_3/Vessel Dynamics1/Vessel LF 6DOF/Rel velocity ==
  note: REL VELOCITY
      | Calculate relative vessel velociy
      | including current.
      | OS2002
  Nu : Inport
  Current : Inport  Port=2
  Mux : Mux  Inputs=2
  Sum : Sum  Inputs=+-  SaturateOnIntegerOverflow=on
  Zeros : Constant  Value=[0 0 0 0]
  Nu_r : Outport
  wires:
  Current/1 -> Mux/1
  Nu/1 -> Sum/1
  Sum/1 -> Nu_r/1
  Mux/1 -> Sum/2
  Zeros/1 -> Mux/2

== system sim_3/Vessel Dynamics1/Vessel LF 6DOF/Rotate_yaw_T ==
  note: ROTATE_YAW_T
      | The transposed rotation matrix in yaw, as defined
      | by Fossen. Rotates a velocity or coordinate a positive
      | yaw angle. Corresponds to matlab function  rotate_yaw_T
      | by OS. Uses the gcn Simulink function GNC: "Transposed
      | rotation matrix yaw"
      | OS2002
  Eta : Inport
  nu_2D_NED : Inport  Port=2
  "GNC: \"Transposed rotation matrix yaw\"" : Subsystem
  Mux : Mux  Inputs=2
  Selector : Selector  InputPortWidth=3  IndexOptions=Index vector (dialog)  Indices=[1 2]  OutputSizes=1
  Selector1 : Selector  InputPortWidth=6  IndexOptions=Index vector (dialog)  Indices=6  OutputSizes=1
  psi : Constant  Value=0
  nu_2D_body : Outport
  wires:
  Selector1/1 -> "GNC: \"Transposed rotation matrix yaw\""/1(psi)
  nu_2D_NED/1 -> Mux/1
  psi/1 -> Mux/2
  "GNC: \"Transposed rotation matrix yaw\""/1(R*nu) -> Selector/1
  Selector/1 -> nu_2D_body/1
  Eta/1 -> Selector1/1
  Mux/1 -> "GNC: \"Transposed rotation matrix yaw\""/2(nu)

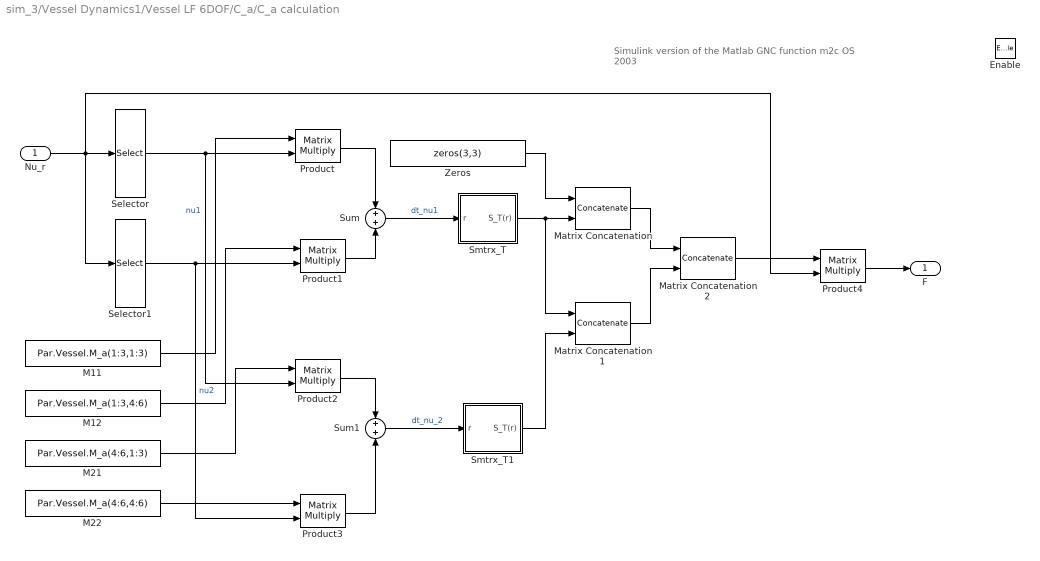
== system sim_3/Vessel Dynamics1/Vessel LF 6DOF/C_a/C_a calculation ==
  note: Simulink version of the Matlab GNC function m2c
      | OS 2003
  Nu_r : Inport
  Enable : EnablePort
  M11 : Constant  Value=Par.Vessel.M_a(1:3,1:3)
  M12 : Constant  Value=Par.Vessel.M_a(1:3,4:6)
  M21 : Constant  Value=Par.Vessel.M_a(4:6,1:3)
  M22 : Constant  Value=Par.Vessel.M_a(4:6,4:6)
  Matrix Concatenation : Concatenate  Mode=Multidimensional array  ConcatenateDimension=2
  Matrix Concatenation1 : Concatenate  Mode=Multidimensional array  ConcatenateDimension=2
  Matrix Concatenation2 : Concatenate  Mode=Multidimensional array
  Product{,1..4} (5 alike) : Product  Multiplication=Matrix(*)  SaturateOnIntegerOverflow=on  OutDataTypeStr=Inherit: Same as first input
  Selector : Selector  InputPortWidth=6  IndexOptions=Index vector (dialog)  Indices=[1:3]  OutputSizes=1
  Selector1 : Selector  InputPortWidth=6  IndexOptions=Index vector (dialog)  Indices=[4:6]  OutputSizes=1
  Smtrx_T : Subsystem
  Smtrx_T1 : Subsystem
  Sum : Sum  Inputs=+|+  SaturateOnIntegerOverflow=on
  Sum1 : Sum  Inputs=+|+  SaturateOnIntegerOverflow=on
  Zeros : Constant  Value=zeros(3,3)
  F : Outport
  wires:
  Nu_r/1 -> Selector/1, Selector1/1, Product4/2
  Product/1 -> Sum/1
  Product1/1 -> Sum/2
  Product2/1 -> Sum1/1
  Product3/1 -> Sum1/2
  Sum/1 -> Smtrx_T/1(r)  "dt_nu1"
  Sum1/1 -> Smtrx_T1/1(r)  "dt_nu_2"
  Zeros/1 -> Matrix Concatenation/1
  Smtrx_T/1(S_T(r)) -> Matrix Concatenation/2, Matrix Concatenation1/1
  Smtrx_T1/1(S_T(r)) -> Matrix Concatenation1/2
  Matrix Concatenation/1 -> Matrix Concatenation2/1
  Matrix Concatenation1/1 -> Matrix Concatenation2/2
  Product4/1 -> F/1
  Selector/1 -> Product/2, Product2/2  "nu1"
  Selector1/1 -> Product1/2, Product3/2  "nu2"
  M11/1 -> Product/1
  M12/1 -> Product1/1
  M22/1 -> Product3/1
  M21/1 -> Product2/1
  Matrix Concatenation2/1 -> Product4/1

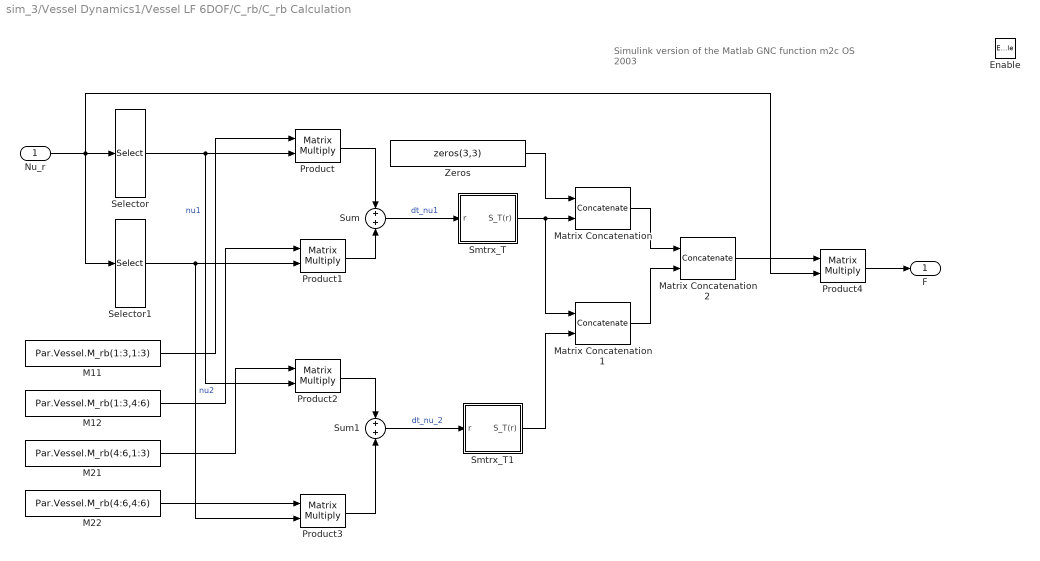
== system sim_3/Vessel Dynamics1/Vessel LF 6DOF/C_rb/C_rb Calculation ==
  note: Simulink version of the Matlab GNC function m2c
      | OS 2003
  Nu_r : Inport
  Enable : EnablePort
  M11 : Constant  Value=Par.Vessel.M_rb(1:3,1:3)
  M12 : Constant  Value=Par.Vessel.M_rb(1:3,4:6)
  M21 : Constant  Value=Par.Vessel.M_rb(4:6,1:3)
  M22 : Constant  Value=Par.Vessel.M_rb(4:6,4:6)
  Matrix Concatenation : Concatenate  Mode=Multidimensional array  ConcatenateDimension=2
  Matrix Concatenation1 : Concatenate  Mode=Multidimensional array  ConcatenateDimension=2
  Matrix Concatenation2 : Concatenate  Mode=Multidimensional array
  Product{,1..4} (5 alike) : Product  Multiplication=Matrix(*)  SaturateOnIntegerOverflow=on  OutDataTypeStr=Inherit: Same as first input
  Selector : Selector  InputPortWidth=6  IndexOptions=Index vector (dialog)  Indices=[1:3]  OutputSizes=1
  Selector1 : Selector  InputPortWidth=6  IndexOptions=Index vector (dialog)  Indices=[4:6]  OutputSizes=1
  Smtrx_T : Subsystem
  Smtrx_T1 : Subsystem
  Sum : Sum  Inputs=+|+  SaturateOnIntegerOverflow=on
  Sum1 : Sum  Inputs=+|+  SaturateOnIntegerOverflow=on
  Zeros : Constant  Value=zeros(3,3)
  F : Outport
  wires:
  Nu_r/1 -> Selector/1, Selector1/1, Product4/2
  Product/1 -> Sum/1
  Product1/1 -> Sum/2
  Product2/1 -> Sum1/1
  Product3/1 -> Sum1/2
  Sum/1 -> Smtrx_T/1(r)  "dt_nu1"
  Sum1/1 -> Smtrx_T1/1(r)  "dt_nu_2"
  Zeros/1 -> Matrix Concatenation/1
  Smtrx_T/1(S_T(r)) -> Matrix Concatenation/2, Matrix Concatenation1/1
  Smtrx_T1/1(S_T(r)) -> Matrix Concatenation1/2
  Matrix Concatenation/1 -> Matrix Concatenation2/1
  Matrix Concatenation1/1 -> Matrix Concatenation2/2
  Product4/1 -> F/1
  Selector/1 -> Product/2, Product2/2  "nu1"
  Selector1/1 -> Product1/2, Product3/2  "nu2"
  M11/1 -> Product/1
  M12/1 -> Product1/1
  M22/1 -> Product3/1
  M21/1 -> Product2/1
  Matrix Concatenation2/1 -> Product4/1

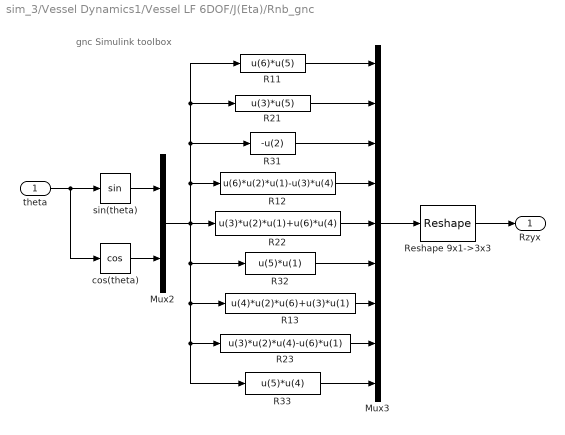
== system sim_3/Vessel Dynamics1/Vessel LF 6DOF/J(Eta)/Rnb_gnc ==
  note: gnc Simulink toolbox
  theta : Inport
  Mux2 : Mux  Inputs=2
  Mux3 : Mux  Inputs=9
  R11 : Fcn  Expr=u(6)*u(5)
  R12 : Fcn  Expr=u(6)*u(2)*u(1)-u(3)*u(4)
  R13 : Fcn  Expr=u(4)*u(2)*u(6)+u(3)*u(1)
  "R21 " : Fcn  Expr=u(3)*u(5)
  R22 : Fcn  Expr=u(3)*u(2)*u(1)+u(6)*u(4)
  R23 : Fcn  Expr=u(3)*u(2)*u(4)-u(6)*u(1)
  "R31 " : Fcn  Expr=-u(2)
  R32 : Fcn  Expr=u(5)*u(1)
  R33 : Fcn  Expr=u(5)*u(4)
  Reshape 9x1->3x3 : Reshape  OutputDimensionality=Customize  OutputDimensions=[3,3]
  cos(theta) : Trigonometry  Operator=cos
  sin(theta) : Trigonometry
  Rzyx : Outport  InitialOutput=0
  wires:
  R11/1 -> Mux3/1
  Mux3/1 -> Reshape 9x1->3x3/1
  Reshape 9x1->3x3/1 -> Rzyx/1
  sin(theta)/1 -> Mux2/1
  cos(theta)/1 -> Mux2/2
  theta/1 -> cos(theta)/1, sin(theta)/1
  Mux2/1 -> R32/1, R13/1, R33/1, R23/1, R22/1, "R31 "/1, R11/1, "R21 "/1, R12/1
  R23/1 -> Mux3/8
  R13/1 -> Mux3/7
  R22/1 -> Mux3/5
  R12/1 -> Mux3/4
  "R31 "/1 -> Mux3/3
  "R21 "/1 -> Mux3/2
  R32/1 -> Mux3/6
  R33/1 -> Mux3/9

== system sim_3/Vessel Dynamics1/Vessel LF 6DOF/J(Eta)/Tnb_gnc ==
  note: gnc Simulink toolbox
  theta : Inport
  Constant : Constant
  "Constant " : Constant  Value=0
  Mux2 : Mux  Inputs=9
  Reshape 9x1->3x3 : Reshape  OutputDimensionality=Customize  OutputDimensions=[3,3]
  "T21 " : Fcn  Expr=sin(u(1))*tan(u(2))
  T22 : Fcn  Expr=cos(u(1))
  T23 : Fcn  Expr=sin(u(1))/cos(u(2))
  "T31 " : Fcn  Expr=cos(u(1))*tan(u(2))
  T32 : Fcn  Expr=-sin(u(1))
  T33 : Fcn  Expr=cos(u(1))/cos(u(2))
  T : Outport  InitialOutput=0
  wires:
  Constant/1 -> Mux2/1
  Mux2/1 -> Reshape 9x1->3x3/1
  Reshape 9x1->3x3/1 -> T/1
  theta/1 -> "T21 "/1, T22/1, "T31 "/1, T32/1, T33/1, T23/1
  T23/1 -> Mux2/6
  T22/1 -> Mux2/5
  T33/1 -> Mux2/9
  "Constant "/1 -> Mux2/2, Mux2/3
  "T21 "/1 -> Mux2/4
  "T31 "/1 -> Mux2/7
  T32/1 -> Mux2/8

== system sim_3/Vessel Dynamics1/Vessel LF 6DOF/Rotate_yaw_T/GNC: "Transposed rotation matrix yaw" ==
  note: GNC: "Transposed
      | rotation matrix yaw"
  psi : Inport
  nu : Inport  Port=2  PortDimensions=3
  Fcn : Fcn  Expr=cos(u(1))*u(2)+sin(u(1))*u(3)
  Fcn1 : Fcn  Expr=-sin(u(1))*u(2)+cos(u(1))*u(3)
  Fcn2 : Fcn  Expr=u(4)
  Mux2 : Mux  Inputs=2
  Mux3 : Mux  Inputs=3
  R*nu : Outport
  wires:
  Mux2/1 -> Fcn1/1, Fcn/1, Fcn2/1
  Fcn/1 -> Mux3/1  "x_dot"
  Fcn1/1 -> Mux3/2  "y_dot"
  Fcn2/1 -> Mux3/3  "psi_dot"
  Mux3/1 -> R*nu/1  "eta_dot"
  psi/1 -> Mux2/1
  nu/1 -> Mux2/2

== system sim_3/Vessel Dynamics1/Vessel LF 6DOF/C_a/C_a calculation/Smtrx_T ==
  note: Transposed S-matrix
  r : Inport
  Mux : Mux  Inputs=9
  Reshape 9x1 => 3x1 : Reshape  OutputDimensionality=Customize  OutputDimensions=[3,3]
  h11 : Fcn  Expr=0
  h12 : Fcn  Expr=u(3)
  h13 : Fcn  Expr=-u(2)
  h21 : Fcn  Expr=-u(3)
  h22 : Fcn  Expr=0
  h23 : Fcn  Expr=u(1)
  h31 : Fcn  Expr=u(2)
  h32 : Fcn  Expr=-u(1)
  h33 : Fcn  Expr=0
  S_T(r) : Outport
  wires:
  r/1 -> h33/1, h23/1, h13/1, h32/1, h22/1, h12/1, h21/1, h11/1, h31/1
  h33/1 -> Mux/9
  h23/1 -> Mux/8
  h13/1 -> Mux/7
  h32/1 -> Mux/6
  h22/1 -> Mux/5
  h12/1 -> Mux/4
  h31/1 -> Mux/3
  h21/1 -> Mux/2
  h11/1 -> Mux/1
  Mux/1 -> Reshape 9x1 => 3x1/1
  Reshape 9x1 => 3x1/1 -> S_T(r)/1

== system sim_3/Vessel Dynamics1/Vessel LF 6DOF/C_a/C_a calculation/Smtrx_T1 ==
  note: Transposed S-matrix
  r : Inport
  Mux : Mux  Inputs=9
  Reshape 9x1 => 3x1 : Reshape  OutputDimensionality=Customize  OutputDimensions=[3,3]
  h11 : Fcn  Expr=0
  h12 : Fcn  Expr=u(3)
  h13 : Fcn  Expr=-u(2)
  h21 : Fcn  Expr=-u(3)
  h22 : Fcn  Expr=0
  h23 : Fcn  Expr=u(1)
  h31 : Fcn  Expr=u(2)
  h32 : Fcn  Expr=-u(1)
  h33 : Fcn  Expr=0
  S_T(r) : Outport
  wires:
  Reshape 9x1 => 3x1/1 -> S_T(r)/1
  Mux/1 -> Reshape 9x1 => 3x1/1
  h11/1 -> Mux/1
  h21/1 -> Mux/2
  h31/1 -> Mux/3
  h12/1 -> Mux/4
  h22/1 -> Mux/5
  h32/1 -> Mux/6
  h13/1 -> Mux/7
  h23/1 -> Mux/8
  h33/1 -> Mux/9
  r/1 -> h31/1, h11/1, h21/1, h12/1, h22/1, h32/1, h13/1, h23/1, h33/1

== system sim_3/Vessel Dynamics1/Vessel LF 6DOF/C_rb/C_rb Calculation/Smtrx_T ==
  note: Transposed S-matrix
  r : Inport
  Mux : Mux  Inputs=9
  Reshape 9x1 => 3x1 : Reshape  OutputDimensionality=Customize  OutputDimensions=[3,3]
  h11 : Fcn  Expr=0
  h12 : Fcn  Expr=u(3)
  h13 : Fcn  Expr=-u(2)
  h21 : Fcn  Expr=-u(3)
  h22 : Fcn  Expr=0
  h23 : Fcn  Expr=u(1)
  h31 : Fcn  Expr=u(2)
  h32 : Fcn  Expr=-u(1)
  h33 : Fcn  Expr=0
  S_T(r) : Outport
  wires:
  r/1 -> h22/1, h12/1, h21/1, h11/1, h31/1, h33/1, h23/1, h13/1, h32/1
  h33/1 -> Mux/9
  h23/1 -> Mux/8
  h13/1 -> Mux/7
  h32/1 -> Mux/6
  h22/1 -> Mux/5
  h12/1 -> Mux/4
  h31/1 -> Mux/3
  h21/1 -> Mux/2
  h11/1 -> Mux/1
  Mux/1 -> Reshape 9x1 => 3x1/1
  Reshape 9x1 => 3x1/1 -> S_T(r)/1

== system sim_3/Vessel Dynamics1/Vessel LF 6DOF/C_rb/C_rb Calculation/Smtrx_T1 ==
  note: Transposed S-matrix
  r : Inport
  Mux : Mux  Inputs=9
  Reshape 9x1 => 3x1 : Reshape  OutputDimensionality=Customize  OutputDimensions=[3,3]
  h11 : Fcn  Expr=0
  h12 : Fcn  Expr=u(3)
  h13 : Fcn  Expr=-u(2)
  h21 : Fcn  Expr=-u(3)
  h22 : Fcn  Expr=0
  h23 : Fcn  Expr=u(1)
  h31 : Fcn  Expr=u(2)
  h32 : Fcn  Expr=-u(1)
  h33 : Fcn  Expr=0
  S_T(r) : Outport
  wires:
  Reshape 9x1 => 3x1/1 -> S_T(r)/1
  Mux/1 -> Reshape 9x1 => 3x1/1
  h11/1 -> Mux/1
  h21/1 -> Mux/2
  h31/1 -> Mux/3
  h12/1 -> Mux/4
  h22/1 -> Mux/5
  h32/1 -> Mux/6
  h13/1 -> Mux/7
  h23/1 -> Mux/8
  h33/1 -> Mux/9
  r/1 -> h31/1, h11/1, h21/1, h12/1, h22/1, h32/1, h13/1, h23/1, h33/1

== matlab function sim_3/Env_force/get wind coefficent  ==
  data: alpha_rw input; C_w output
function C_w   = getC_w(alpha_rw)


C_wind =    [248.37 0 0 0 -2355.232759 0;
            265.19 61.332 0 275.994 -2514.732759 551.1;
            224.13 136.22 0 612.99 -2125.37069 661.56;
            149.03 238.76 0 1074.42 -1413.215517 451.37;
            134.36 319.42 0 1437.39 -1274.103448 212.51;
            96.8 380.5 0 1712.25 -917.9310345 -23.578;
            41.364 396.1 0 1782.45 -392.2448276 1168.3;
            16.477 372.96 0 1678.32 -156.2474138 2376.3;
            0.30412 376.5 0 1694.25 -2.883896552 3511.9;
            -3.723 390.01 0 1755.045 35.30431034 4610.4;
            -24.879 386.63 0 1739.835 235.9215517 4769.5;
            -61.281 393.76 0 1771.92 581.112931 5921.9;
            -108.5 408.66 0 1838.97 1028.87931 6542.8;
            -169.35 393.26 0 1769.67 1605.905172 6805.2;    
            -206.63 276.93 0 1246.185 1959.422414 6751.5;
            -201.99 200.64 0 902.88 1915.422414 6190.1;
            -196.51 124.71 0 561.195 1863.456897 3758.8;
            -181.53 56.27 0 253.215 1721.405172 1905.6;
            -208.22 0 0 0 1974.5 0;
            -181.53 -56.27 0 -253.215 1721.405172 -1905.6;
            -196.51 -124.71 0 -561.195 1863.456897 -3758.8;
            -201.99 -200.64 0 -902.88 1915.422414 -6190.1;
            -206.63 -276.93 0 -1246.185 1959.422414 -6751.5;
            -169.35 -393.26 0 -1769.67 1605.905172 -6805.2;
            -108.5 -408.66 0 -1838.97 1028.87931 -6542.8;
            -61.281 -393.76 0 -1771.92 581.112931 -5921.9;
            -24.879 -386.63 0 -1739.835 235.9215517 -4769.5;
            -3.723 -390.01 0 -1755.045 35.30431034 -4610.4;
            0.30412 -376.5 0 -1694.25 -2.883896552 -3511.9;
            16.477 -372.96 0 -1678.32 -156.2474138 -2376.3;
            41.364 -396.1 0 -1782.45 -392.2448276 -1168.3;
            96.8 -380.5 0 -1712.25 -917.9310345 23.578;
            134.36 -319.42 0 -1437.39 -1274.103448 -212.51;
            149.03 -238.76 0 -1074.42 -1413.215517 -451.37;
            224.13 -136.22 0 -612.99 -2125.37069 -661.56;
            265.19 -61.332 0 -275.994 -2514.732759 -551.1;
            248.37 0 0 0 -2355.232759 0;];
        


% Get alpha between 0 -360
while alpha_rw > 360
    alpha_rw = alpha_rw - 360;
end

while alpha_rw < 0
    alpha_rw = alpha_rw + 360;
end

avrundet_alpha = alpha_rw - mod(alpha_rw,10);
index = avrundet_alpha/10+1;

C_w= C_wind(index,:)';
end

== matlab function sim_3/Env_force/get current coefficent  ==
  data: alpha_rc input; C_c output
function C_c   = getC_c(alpha_rc)

C_current = [11786 0 0 0 33000.8 0;
            13751 24354 0 -68191.2 38502.8 -571850;
            15322 46496 0 -130188.8 42901.6 -947490;
            16304 70808 0 -198262.4 45651.2 -1270900;
            16304 95206 0 -266576.8 45651.2 -1501300;
            14339 121710 0 -340788 40149.2 -1447700;
            11000 146070 0 -408996 30800 -1179900;
            7268.3 164050 0 -459340 20351.24 -858400;
            3143 174920 0 -489776 8800.4 -500840;
            -1374.8 179300 0 -502040 -3849.44 -107140;
            -5107.6 174850 0 -489580 -14301.28 214290;
            -8839.1 166060 0 -464968 -24749.48 518280;
            -11982 150570 0 -421596 -33549.6 607860;
            -14339 126300 0 -353640 -40149.2 947490;
            -14537 97417 0 -272767.6 -40703.6 947490;
            -12376 68636 0 -192180.8 -34652.8 750880;
            -10410 42066 0 -117784.8 -29148 518470;
            -9427.9 19898 0 -55714.4 -26398.12 249180;
            -9231.9 0 0 0 -25849.32 0;
            -9427.9 -19898 0 55714.4 -26398.12 -249180
            -10410 -42066 0 117784.8 -29148 -518470;
            -12376 -68636 0 192180.8 -34652.8 -750880;
            -14537 -97417 0 272767.6 -40703.6 -947490;
            -14339 -126300 0 353640 -40149.2 -947490;
            -11982 -150570 0 421596 -33549.6 -607860;
            -8839.1 -166060 0 464968 -24749.48 -518280;
            -5107.6 -174850 0 489580 -14301.28 -214290;
            -1374.8 -179300 0 502040 -3849.44 107140;
            3143 -174920 0 489776 8800.4 500840;
            7268.3 -164050 0 459340 20351.24 858400;
            11000 -146070 0 408996 30800 1179900;
            14339 -121710 0 340788 40149.2 1447700;
            16304 -95206 0 266576.8 45651.2 1501300;
            16304 -70808 0 198262.4 45651.2 1270900;
            15322 -46496 0 130188.8 42901.6 947490;
            13751 -24354 0 68191.2 38502.8 571850;
            11786 0 0 0 33000.8 0;];
        


% Get alpha between 0 -360
while alpha_rc > 360
    alpha_rc = alpha_rc - 360;
end

while alpha_rc < 0
    alpha_rc = alpha_rc + 360;
end

avrundet_alpha = alpha_rc - mod(alpha_rc,10);
index = avrundet_alpha/10+1;

C_c= C_current(index,:)';
end

== matlab function sim_3/Env_NEW/Wind/Slowly-varying wind + gust/by using Harris Spectrum ==
  data: S input; Ug output; f input; phi input; N_freq input; t input
function Ug = fcn(S, f, phi, N_freq, t)
Ug = 0; % dummy value due to Ug first defined in for-loop
for i = 1:N_freq
    Ug = Ug + sqrt(2*S(i)*(f(2)-f(1))) * cos(2*pi*f(i)*t + phi(i));
end
end

== matlab function sim_3/Env_NEW/get current coeffcients ==
  data: alpha input; C output; currentCoeffMatrix input
function C   = CurrentCoefficients( alpha, currentCoeffMatrix )
% Initialization of the return parameter
C=zeros(6,1);

while alpha > 360
    alpha = alpha - 360;
end

while alpha < 0
    alpha = alpha + 360;
end

alpha_mod = mod(alpha,10);
avrundet_alpha = alpha - alpha_mod;
index = avrundet_alpha/10+1;

C1 = currentCoeffMatrix(index,:)';
C2 = currentCoeffMatrix(index+1,:)';

for i = 1:6
    diff = C2(i)-C1(i);
    point = (diff/10)*alpha_mod;
    C(i) = C1(i)+point;
end

end

== matlab function sim_3/Env_NEW/get wind coeffcients ==
  data: alpha input; C output; windCoeffMatrix input
function C   = WindCoeffcients(alpha, windCoeffMatrix)
% Initialization of the return parameter
C=zeros(6,1);

while alpha > 360
    alpha = alpha - 360;
end

while alpha < 0
    alpha = alpha + 360;
end

alpha_mod = mod(alpha,10);
avrundet_alpha = alpha - alpha_mod;
index = avrundet_alpha/10+1;

C1 = windCoeffMatrix(index,:)';
C2 = windCoeffMatrix(index+1,:)';

for i = 1:6
    diff = C2(i)-C1(i);
    point = (diff/10)*alpha_mod;
    C(i) = C1(i)+point;
end

end
